simulink model "Microphone_Model"  (R2019b)
settings: Solver=VariableStepAuto  StartTime=0.0  StopTime=33  RelTol=1e-6
InitFcn:
  | F = 1e-4; v=48e-4; i0=3e-3;
  | m=50e-3; K=1e-1;
  | D = 3e-5; Bl=0.5;
  | R = 5; L=45;
settings Model: Creator=sulaymon.eshkabilov  LastModifiedBy=sulaymon.eshkabilov

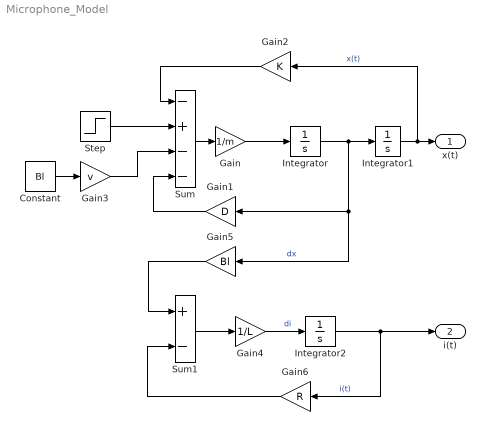
== system Microphone_Model ==
  Constant : Constant  Value=Bl
  Gain : Gain  Gain=1/m
  Gain1 : Gain  Gain=D
  Gain2 : Gain  Gain=K
  Gain3 : Gain  Gain=v
  Gain4 : Gain  Gain=1/L
  Gain5 : Gain  Gain=Bl
  Gain6 : Gain  Gain=R
  Integrator : Integrator
  Integrator1 : Integrator
  Integrator2 : Integrator  InitialCondition=i0
  Step : Step  Time=v  SampleTime=0
  Sum : Sum  Inputs=-+--
  Sum1 : Sum  Inputs=+-
  x(t) : Outport
  i(t) : Outport  Port=2
  wires:
  Integrator/1 -> Integrator1/1, Gain5/1, Gain1/1  "dx"
  Sum/1 -> Gain/1
  Sum1/1 -> Gain4/1
  Gain/1 -> Integrator/1
  Integrator1/1 -> x(t)/1, Gain2/1  "x(t)"
  Step/1 -> Sum/2
  Constant/1 -> Gain3/1
  Gain3/1 -> Sum/3
  Gain4/1 -> Integrator2/1  "di"
  Gain5/1 -> Sum1/1
  Integrator2/1 -> i(t)/1, Gain6/1  "i(t)"
  Gain6/1 -> Sum1/2
  Gain2/1 -> Sum/1
  Gain1/1 -> Sum/4
